simulink model "Simulation_Example_v2"  (R2017b)
settings: Solver=VariableStepAuto  StartTime=0.0  StopTime=100  RelTol=1e-3
libraries: SY202_NCS_Library x9
settings Model: Creator=rodrigue  LastModifiedBy=rodrigue

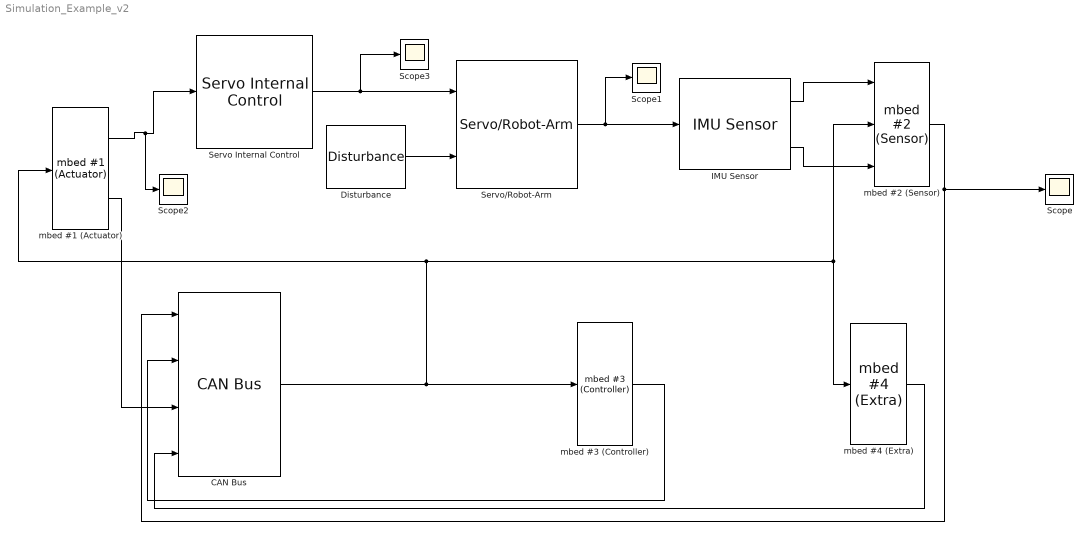
== system Simulation_Example_v2 ==
  CAN Bus : SY202_NCS_Library/CAN Bus
  Disturbance : SY202_NCS_Library/Disturbance  DisturbanceTime=20  DisturbanceValue=0
  IMU Sensor : SY202_NCS_Library/IMU Sensor  MeanSensorError=0  MeanSensorVar=0.001
  Scope{,1..3} (4 alike) : Scope
  Servo Internal Control : SY202_NCS_Library/Servo Internal Control  MaxPW=2100  MinPW=900  MaxServo=pi/3  MinServo=-pi/3
  Servo/Robot-Arm : SY202_NCS_Library/Servo//Robot-Arm  x0=-.5  xdot0=0  MaxPW=2100  MinPW=900  MaxServo=pi/3  MinServo=-pi/3
  mbed #1 (Actuator) : SY202_NCS_Library/mbed #1 (Actuator)  MinPW=900  MaxPW=2100
  mbed #2 (Sensor) : SY202_NCS_Library/mbed #2 (Sensor)
  mbed #3 (Controller) : SY202_NCS_Library/mbed #3 (Controller)  DesValue=0  Kp=100  Ki=300  Offset=1400
  mbed #4 (Extra) : SY202_NCS_Library/mbed #4 (Extra)  AttackRate=50  AttackMode=Replay Attack (Variant)  AttackMag=0.4  AttackTime=20
  wires:
  mbed #2 (Sensor)/1 -> Scope/1, CAN Bus/1
  mbed #1 (Actuator)/1 -> Servo Internal Control/1, Scope2/1
  Servo Internal Control/1 -> Scope3/1, Servo/Robot-Arm/1
  Disturbance/1 -> Servo/Robot-Arm/2
  Servo/Robot-Arm/1 -> Scope1/1, IMU Sensor/1
  IMU Sensor/1 -> mbed #2 (Sensor)/1
  IMU Sensor/2 -> mbed #2 (Sensor)/3
  mbed #1 (Actuator)/2 -> CAN Bus/3
  mbed #3 (Controller)/1 -> CAN Bus/2
  mbed #4 (Extra)/1 -> CAN Bus/4
  CAN Bus/1 -> mbed #4 (Extra)/1, mbed #2 (Sensor)/2, mbed #1 (Actuator)/1, mbed #3 (Controller)/1
